simulink model "autonomous_system"  (R2020b)
settings: Solver=FixedStepAuto  StartTime=0.0  StopTime=10.0  FixedStep=1e-4  RelTol=1e-3
model workspace (MAT data in the model file):
  theta_dot = 0
settings Model: Creator=avina  LastModifiedBy=avina

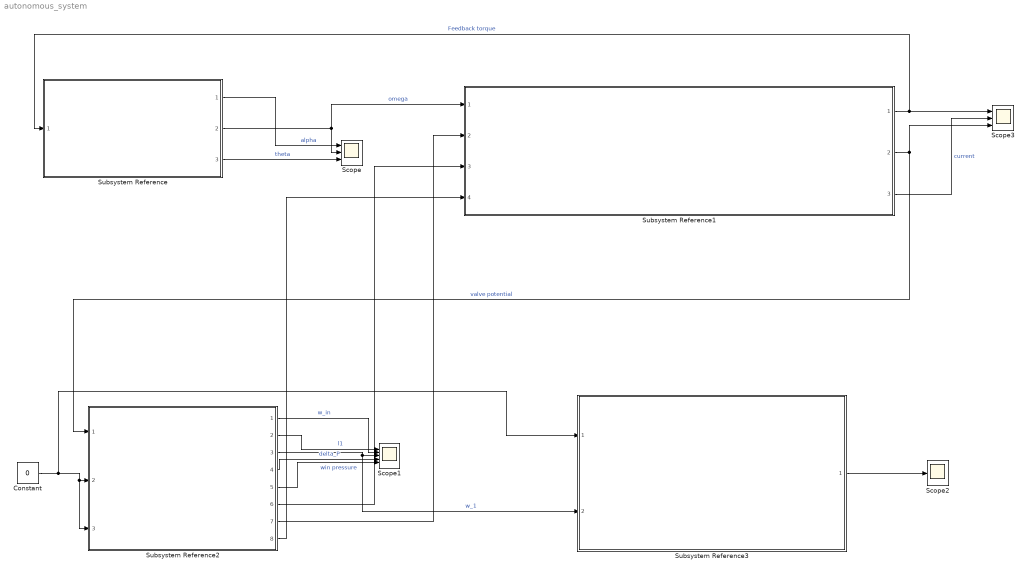
== system autonomous_system ==
  Constant : Constant  Value=0
  Scope : Scope  NumInputPorts=3
  Scope1 : Scope  NumInputPorts=5
  Scope2 : Scope
  Scope3 : Scope  NumInputPorts=3
  Subsystem Reference : Subsystem  ReferencedSubsystem=Pendulum
  Subsystem Reference1 : Subsystem  ReferencedSubsystem=Motor_circuit
  Subsystem Reference2 : Subsystem  ReferencedSubsystem=Tank_system
  Subsystem Reference3 : Subsystem  ReferencedSubsystem=Dissipator_circuit
  wires:
  Subsystem Reference/2 -> Scope/2, Subsystem Reference1/1  "omega"
  Subsystem Reference1/1 -> Subsystem Reference/1, Scope3/1  "Feedback torque"
  Subsystem Reference1/2 -> Scope3/3, Subsystem Reference2/1  "valve potential"
  Subsystem Reference2/4 -> Scope1/4  "delta_P"
  Subsystem Reference2/1 -> Scope1/2  "w_in"
  Subsystem Reference2/3 -> Subsystem Reference3/2, Scope1/3  "w_1"
  Constant/1 -> Subsystem Reference2/2, Subsystem Reference2/3, Subsystem Reference3/1
  Subsystem Reference/1 -> Scope/1  "alpha"
  Subsystem Reference/3 -> Scope/3  "theta"
  Subsystem Reference2/2 -> Scope1/1  "l1"
  Subsystem Reference3/1 -> Scope2/1
  Subsystem Reference1/3 -> Scope3/2  "current"
  Subsystem Reference2/5 -> Scope1/5  "win pressure"
  Subsystem Reference2/6 -> Subsystem Reference1/3
  Subsystem Reference2/7 -> Subsystem Reference1/2
  Subsystem Reference2/8 -> Subsystem Reference1/4
